simulink model "modelo_robot_3dof_dininv"  (R2023b)
settings: Solver=ode5  StartTime=0.0  StopTime=tsim  FixedStep=tstep  RelTol=1e-3
undefined symbols (not defined in the file): robot_params
settings Model: Creator=HP  LastModifiedBy=HP

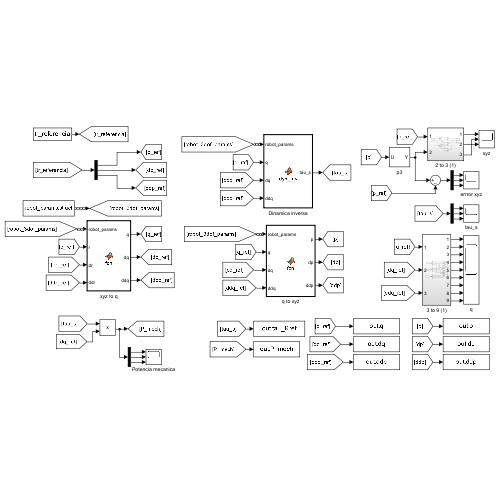
[thumbnail: Simulink's stored preview of the top-level diagram]
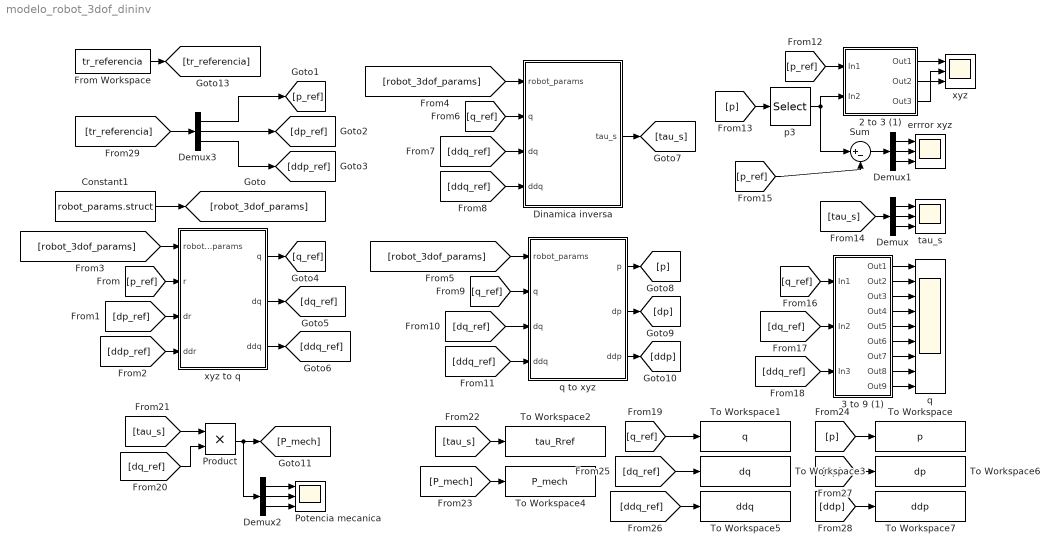
== system modelo_robot_3dof_dininv ==
  2 to 3 (1) : Subsystem
  3 to 9 (1) : Subsystem
  Constant1 : Constant  Value=robot_params.struct  OutDataTypeStr=Bus: robot_params_bus
  Demux{,1..3} (4 alike) : Demux  Outputs=3
  Dinamica inversa : MATLAB Function  TreatAsAtomicUnit=on
  From Workspace : FromWorkspace  VariableName=tr_referencia
  Potencia mecanica : Scope  NumInputPorts=3
  Product : Product
  Sum : Sum  Inputs=|+-
  To Workspace : ToWorkspace  VariableName=p  SaveFormat=Timeseries  SampleTime=-1
  To Workspace1 : ToWorkspace  VariableName=q  SaveFormat=Timeseries  SampleTime=-1
  To Workspace2 : ToWorkspace  VariableName=tau_Rref  SaveFormat=Timeseries  SampleTime=-1
  To Workspace3 : ToWorkspace  VariableName=dq  SaveFormat=Timeseries  SampleTime=-1
  To Workspace4 : ToWorkspace  VariableName=P_mech  SaveFormat=Timeseries  SampleTime=-1
  To Workspace5 : ToWorkspace  VariableName=ddq  SaveFormat=Timeseries  SampleTime=-1
  To Workspace6 : ToWorkspace  VariableName=dp  SaveFormat=Timeseries  SampleTime=-1
  To Workspace7 : ToWorkspace  VariableName=ddp  SaveFormat=Timeseries  SampleTime=-1
  errror xyz : Scope  NumInputPorts=3
  p3 : Selector  NumberOfDimensions=2  InputPortWidth=3  IndexOptions=Index vector (dialog),Index vector (dialog)  Indices=[1:3],3  OutputSizes=1,1
  q : Scope  NumInputPorts=9
  q to xyz : MATLAB Function  TreatAsAtomicUnit=on
  tau_s : Scope  NumInputPorts=3
  xyz : Scope  NumInputPorts=3
  xyz to q : MATLAB Function  TreatAsAtomicUnit=on
  wires:
  Constant1/1 -> [robot_3dof_params]
  [robot_3dof_params] -> xyz to q/1(robot_params)
  [robot_3dof_params] -> Dinamica inversa/1(robot_params)
  [robot_3dof_params] -> q to xyz/1(robot_params)
  [p_ref] -> xyz to q/2(r)
  [dp_ref] -> xyz to q/3(dr)
  [ddp_ref] -> xyz to q/4(ddr)
  xyz to q/1(q) -> [q_ref]
  xyz to q/2(dq) -> [dq_ref]
  xyz to q/3(ddq) -> [ddq_ref]
  [q_ref] -> Dinamica inversa/2(q)
  [ddq_ref] -> Dinamica inversa/3(dq)
  [ddq_ref] -> Dinamica inversa/4(ddq)
  [q_ref] -> q to xyz/2(q)
  [dq_ref] -> q to xyz/3(dq)
  [ddq_ref] -> q to xyz/4(ddq)
  Dinamica inversa/1(tau_s) -> [tau_s]
  q to xyz/1(p) -> [p]
  q to xyz/3(ddp) -> [ddp]
  q to xyz/2(dp) -> [dp]
  [p_ref] -> 2 to 3 (1)/1(In1)
  2 to 3 (1)/1(Out1) -> xyz/1
  2 to 3 (1)/2(Out2) -> xyz/2
  2 to 3 (1)/3(Out3) -> xyz/3
  [tau_s] -> Demux/1
  Demux/1 -> tau_s/1
  Demux/2 -> tau_s/2
  Demux/3 -> tau_s/3
  [p] -> p3/1
  [p_ref] -> Sum/2
  Sum/1 -> Demux1/1
  Demux1/1 -> errror xyz/1
  Demux1/2 -> errror xyz/2
  Demux1/3 -> errror xyz/3
  p3/1 -> Sum/1, 2 to 3 (1)/2(In2)
  [q_ref] -> 3 to 9 (1)/1(In1)
  [dq_ref] -> 3 to 9 (1)/2(In2)
  [ddq_ref] -> 3 to 9 (1)/3(In3)
  3 to 9 (1)/1(Out1) -> q/1
  3 to 9 (1)/2(Out2) -> q/2
  3 to 9 (1)/3(Out3) -> q/3
  3 to 9 (1)/4(Out4) -> q/4
  3 to 9 (1)/5(Out5) -> q/5
  3 to 9 (1)/6(Out6) -> q/6
  3 to 9 (1)/7(Out7) -> q/7
  3 to 9 (1)/8(Out8) -> q/8
  3 to 9 (1)/9(Out9) -> q/9
  [tau_s] -> Product/1
  [dq_ref] -> Product/2
  [q_ref] -> To Workspace1/1
  [tau_s] -> To Workspace2/1
  Product/1 -> Demux2/1, [P_mech]
  [P_mech] -> To Workspace4/1
  [p] -> To Workspace/1
  Demux2/1 -> Potencia mecanica/1
  Demux2/2 -> Potencia mecanica/2
  Demux2/3 -> Potencia mecanica/3
  [dq_ref] -> To Workspace3/1
  [ddq_ref] -> To Workspace5/1
  [dp] -> To Workspace6/1
  [ddp] -> To Workspace7/1
  [tr_referencia] -> Demux3/1
  From Workspace/1 -> [tr_referencia]
  Demux3/1 -> [p_ref]
  Demux3/2 -> [dp_ref]
  Demux3/3 -> [ddp_ref]

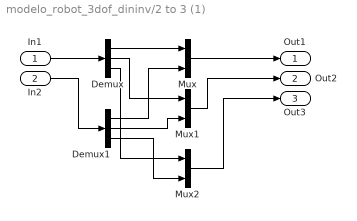
== system modelo_robot_3dof_dininv/2 to 3 (1) ==
  In1 : Inport
  In2 : Inport  Port=2
  Demux : Demux  Outputs=3
  Demux1 : Demux  Outputs=3
  Mux : Mux  Inputs=2
  Mux1 : Mux  Inputs=2
  Mux2 : Mux  Inputs=2
  Out1 : Outport
  Out2 : Outport  Port=2
  Out3 : Outport  Port=3
  wires:
  Demux/3 -> Mux2/1
  Mux2/1 -> Out3/1
  Mux1/1 -> Out2/1
  Demux/1 -> Mux/1
  Demux1/1 -> Mux/2
  In1/1 -> Demux/1
  Demux/2 -> Mux1/1
  Demux1/2 -> Mux1/2
  Mux/1 -> Out1/1
  Demux1/3 -> Mux2/2
  In2/1 -> Demux1/1

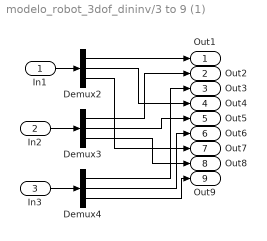
== system modelo_robot_3dof_dininv/3 to 9 (1) ==
  In1 : Inport
  In2 : Inport  Port=2
  In3 : Inport  Port=3
  Demux2 : Demux  Outputs=3
  Demux3 : Demux  Outputs=3
  Demux4 : Demux  Outputs=3
  Out1 : Outport
  Out2 : Outport  Port=2
  Out3 : Outport  Port=3
  Out4 : Outport  Port=4
  Out5 : Outport  Port=5
  Out6 : Outport  Port=6
  Out7 : Outport  Port=7
  Out8 : Outport  Port=8
  Out9 : Outport  Port=9
  wires:
  In3/1 -> Demux4/1
  Demux4/1 -> Out3/1
  Demux2/1 -> Out1/1
  Demux3/3 -> Out8/1
  Demux3/2 -> Out5/1
  Demux3/1 -> Out2/1
  In1/1 -> Demux2/1
  Demux2/3 -> Out7/1
  Demux4/3 -> Out9/1
  Demux4/2 -> Out6/1
  Demux2/2 -> Out4/1
  In2/1 -> Demux3/1

== matlab function modelo_robot_3dof_dininv/xyz to q ==
  data: robot_params input; q output size=[3,1]; r input size=[3,1]; dr input size=[3,1]; ddr input size=[3,1]; dq output size=[3,1]; ddq output size=[3,1]
function [q,dq,ddq] = fcn(robot_params,r,dr,ddr)

d1 = robot_params.d(1);
l2 = robot_params.l(2);
l3 = robot_params.l(3);

Xr = r(1);
Yr = r(2);
Zr = r(3);


c3 = (Xr^2+Yr^2+(Zr-d1)^2-l2^2-l3^2)/(2*l2*l3);

q1 = atan2(Yr,Xr);
q2 = atan2(Zr-d1,sqrt(Xr^2+Yr^2)) - atan2(-l3*sqrt(1-c3^2),l2+l3*c3);
q3 = atan2(-sqrt(1-c3^2),c3);

q = [q1;q2;q3];

JPinv = zeros(3,3);
JPinv(1,1) = -sin(q1)/(l2*cos(q2) + l3*cos(q2 + q3));
JPinv(1,2) = cos(q1)/(l2*cos(q2) + l3*cos(q2 + q3));

JPinv(2,1) = cos(q1)*cos(q2 + q3)/(l2*sin(q3));
JPinv(2,2) = sin(q1)*cos(q2 + q3)/(l2*sin(q3));
JPinv(2,3) = sin(q2 + q3)/(l2*sin(q3));

JPinv(3,1) = -(cos(q1)*(l2*cos(q2) + l3*cos(q2 + q3)))/(l2*l3*sin(q3));
JPinv(3,2) = -(sin(q1)*(l2*cos(q2) + l3*cos(q2 + q3)))/(l2*l3*sin(q3));
JPinv(3,3) = -(l2*sin(q2) + l3*sin(q2 + q3))/(l2*l3*sin(q3));

dq = JPinv*dr;

dq1 = dq(1);
dq2 = dq(2);
dq3 = dq(3);


dJP = zeros(3,3);

dJP(1,1) = - cos(q1)*(l2*cos(q2) + l3*cos(q2 + q3))*dq1 + sin(q1)*(l2*sin(q2) + l3*sin(q2 + q3))*dq2 + l3*sin(q1)*sin(q2 + q3)*dq3;
dJP(1,2) =   sin(q1)*(l2*sin(q2) + l3*sin(q2 + q3))*dq1 - cos(q1)*(l2*cos(q2) + l3*cos(q2 + q3))*dq2 - l3*cos(q1)*cos(q2 + q3)*dq3;
dJP(1,3) =   l3*sin(q1)*sin(q2 + q3)*dq1 - l3*cos(q1)*cos(q2 + q3)*dq2 - l3*cos(q1)*cos(q2 + q3)*dq3;

dJP(2,1) = - sin(q1)*(l2*cos(q2) + l3*cos(q2 + q3))*dq1 - cos(q1)*(l2*sin(q2) + l3*sin(q2 + q3))*dq2 - l3*cos(q1)*sin(q2 + q3)*dq3;
dJP(2,2) = - cos(q1)*(l2*sin(q2) + l3*sin(q2 + q3))*dq1 - sin(q1)*(l2*cos(q2) + l3*cos(q2 + q3))*dq2 - l3*sin(q1)*cos(q2 + q3)*dq3;
dJP(2,3) = - l3*cos(q1)*sin(q2 + q3)*dq1 - l3*sin(q1)*cos(q2 + q3)*dq2 - l3*sin(q1)*cos(q2 + q3)*dq3;

dJP(3,1) = 0;
dJP(3,2) = - (l2*sin(q2) + l3*sin(q2 + q3))*dq2 - l3*sin(q2 + q3)*dq3;
dJP(3,3) = - l3*sin(q2 + q3)*(dq2 + dq3);

ddq = JPinv*(ddr - dJP*dq);

== matlab function modelo_robot_3dof_dininv/q to xyz ==
  data: robot_params input; p output size=[3,3]; q input size=[3,1]; dq input size=[3,1]; ddq input size=[3,1]; dp output size=[3,1]; ddp output size=[3,1]
function [p,dp,ddp] = fcn(robot_params,q,dq,ddq)

d1 = robot_params.d(1);
l2 = robot_params.l(2);
l3 = robot_params.l(3);

q1 = q(1);
q2 = q(2);
q3 = q(3);

p1 = [0;0;d1];

p2 = [l2*cos(q1)*cos(q2);
      l2*sin(q1)*cos(q2);
      d1+l2*sin(q2)];

p3 = [cos(q1)*(l2*cos(q2)+l3*cos(q2+q3));
      sin(q1)*(l2*cos(q2)+l3*cos(q2+q3));
      d1+l2*sin(q2)+l3*sin(q2+q3)];

p = [p1,p2,p3];

JP = zeros(3,3);

JP(1,1) = -sin(q1)*(l2*cos(q2) + l3*cos(q2 + q3));
JP(1,2) = -cos(q1)*(l2*sin(q2) + l3*sin(q2 + q3));
JP(1,3) = -l3*cos(q1)*sin(q2 + q3);

JP(2,1) =  cos(q1)*(l2*cos(q2) + l3*cos(q2 + q3));
JP(2,2) = -sin(q1)*(l2*sin(q2) + l3*sin(q2 + q3));
JP(2,3) = -l3*sin(q1)*sin(q2 + q3);

JP(3,2) = l2*cos(q2) + l3*cos(q2 + q3);
JP(3,3) = l3*cos(q2 + q3);

dp = JP*dq;
dq1 = dq(1);
dq2 = dq(2);
dq3 = dq(3);

dJ = zeros(3,3);

dJ(1,1) = - cos(q1)*(l2*cos(q2) + l3*cos(q2 + q3))*dq1 + sin(q1)*(l2*sin(q2) + l3*sin(q2 + q3))*dq2 + l3*sin(q1)*sin(q2 + q3)*dq3;
dJ(1,2) =   sin(q1)*(l2*sin(q2) + l3*sin(q2 + q3))*dq1 - cos(q1)*(l2*cos(q2) + l3*cos(q2 + q3))*dq2 - l3*cos(q1)*cos(q2 + q3)*dq3;
dJ(1,3) =   l3*sin(q1)*sin(q2 + q3)*dq1 - l3*cos(q1)*cos(q2 + q3)*dq2 - l3*cos(q1)*cos(q2 + q3)*dq3;

dJ(2,1) = - sin(q1)*(l2*cos(q2) + l3*cos(q2 + q3))*dq1 - cos(q1)*(l2*sin(q2) + l3*sin(q2 + q3))*dq2 - l3*cos(q1)*sin(q2 + q3)*dq3;
dJ(2,2) = - cos(q1)*(l2*sin(q2) + l3*sin(q2 + q3))*dq1 - sin(q1)*(l2*cos(q2) + l3*cos(q2 + q3))*dq2 - l3*sin(q1)*cos(q2 + q3)*dq3;
dJ(2,3) = - l3*cos(q1)*sin(q2 + q3)*dq1 - l3*sin(q1)*cos(q2 + q3)*dq2 - l3*sin(q1)*cos(q2 + q3)*dq3;

dJ(3,1) = 0;
dJ(3,2) = - (l2*sin(q2) + l3*sin(q2 + q3))*dq2 - l3*sin(q2 + q3)*dq3;
dJ(3,3) = - l3*sin(q2 + q3)*(dq2 + dq3);

ddp = dJ*ddq;

== matlab function modelo_robot_3dof_dininv/Dinamica inversa ==
  data: robot_params input; q input size=[3,1]; tau_s output size=[3,1]; dq input size=[3,1]; ddq input size=[3,1]
function tau_s = dyn_inv(robot_params,q,dq,ddq)

%d1 = robot_params.d(1);
l2 = robot_params.l(2);
lc2 = robot_params.lc(2);
%l3 = robot_params.l(3);
lc3 = robot_params.lc(3);

%m1 = robot_params.m(1);
m2 = robot_params.m(2);
m3 = robot_params.m(3);

Iz1 = robot_params.I(1,3);
Iy2 = robot_params.I(2,2);
Iz2 = robot_params.I(2,3);
Iy3 = robot_params.I(3,2);
Iz3 = robot_params.I(3,3);

g = 9.81;

q1 = q(1);
q2 = q(2);
q3 = q(3);

dq1 = dq(1);
dq2 = dq(2);
dq3 = dq(3);

D = zeros(3,3);

D(1,1) = Iz1 + Iz2 + Iz3 + (m2/2)*lc2^2*(1+cos(2*q2)) ...
       + (m3/2)*(l2^2*(1+cos(2*q2)) + 2*l2*lc3*(cos(2*q2+q3)+cos(q3)) ...
       + lc3^2*(1+cos(2*q2+2*q3)));

D(2,2) = Iy2 + Iy3 + m2*lc2^2 + m3*(l2^2 + 2*l2*lc3*cos(q3) + lc3^2);
D(2,3) = Iy3 + m3*(l2*lc3*cos(q3) + lc3^2);

D(3,2) = Iy3 + m3*(l2*lc3*cos(q3) + lc3^2);
D(3,3) = Iy3 + m3*lc3^2;

C = zeros(3,3);

C(1,2) = - ((m2*lc2^2*sin(2*q2)) ...
         + m3*(l2^2*sin(2*q2) + 2*l2*lc3*sin(2*q2+q3) ...
         + lc3^2*sin(2*q2+2*q3)))*dq1;
C(1,3) = - m3*(l2*lc3*(sin(2*q2+q3)+sin(q3)) ...
         + lc3^2*(sin(2*q2+2*q3)))*dq1;

C(2,1) =   ((m2/2)*(lc2^2*sin(2*q2)) ...
         + (m3/2)*(l2^2*sin(2*q2) + 2*l2*lc3*sin(2*q2+q3) ...
         + lc3^2*sin(2*q2+2*q3)))*dq1;
C(2,2) = - 2*m3*l2*lc3*sin(q3)*dq3;
C(2,3) = - m3*l2*lc3*sin(q3)*dq3;

C(3,1) =   (m3/2)*(l2*lc3*(sin(2*q2+q3) + sin(q3)) ...
         + lc3^2*sin(2*q2+2*q3))*dq1;
C(3,2) =   m3*l2*lc3*sin(q3)*dq2;

G = zeros(3,1);

G(2,1) = m2*lc2*cos(q2) + m3*(l2*cos(q2) + lc3*cos(q2+q3));
G(3,1) = m3*lc3*cos(q2+q3);


tau_s = D*ddq + C*dq + G*g;
